simulink model "MBD_W3_Prob3"  (R2020a)
settings: Solver=ode45  StartTime=0.0  StopTime=25  MaxStep=0.01  RelTol=1e-3  AbsTol=1e-6
values from neighbouring files (symbols this model uses):
  g = 9.81    [Prob3.m]
  I = 5    [Prob3.m]
  Kf = 1    [Prob3.m]
  m = 75    [Prob3.m]
  mu = [0 .4 .8 .97 1.0 .98 .96 .94 .92 .9 .88 .855 .83 .81 .79 .77 .75 .73 .72 .71 .7]    [Prob3.m]
  PBmax = 1500    [Prob3.m]
  Rr = 15/12    (= 1.25)    [Prob3.m]
  slip = (0:.05:1.0)    [Prob3.m]
  TB = 0.01    [Prob3.m]
  v0 = 45    [Prob3.m]
settings Model: Creator=Noel Varghese  LastModifiedBy=Noel Varghese

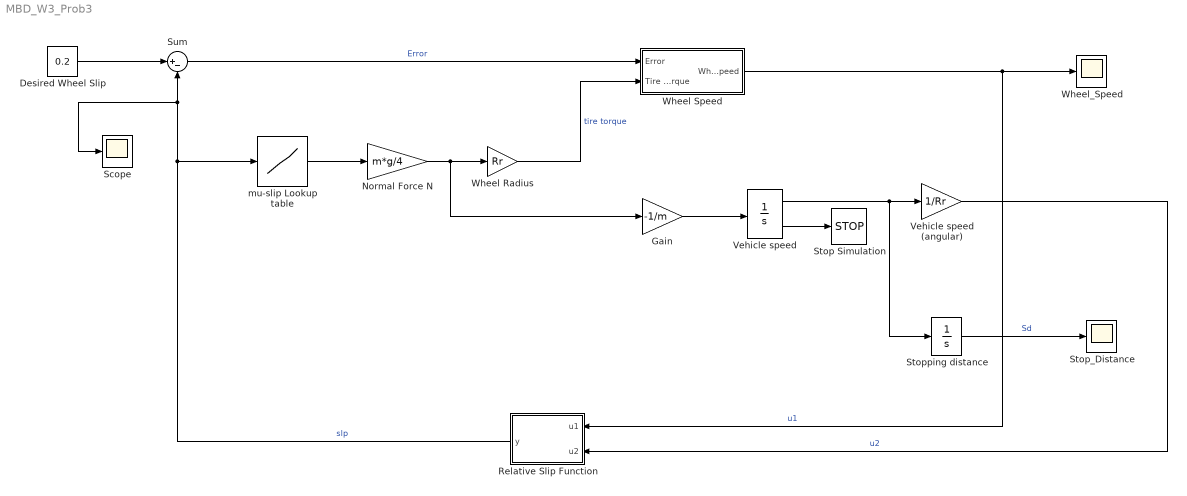
== system MBD_W3_Prob3 ==
  Desired Wheel Slip : Constant  Value=0.2
  Gain : Gain  Gain=-1/m
  Normal Force N : Gain  Gain=m*g/4
  Relative Slip Function : MATLAB Function  TreatAsAtomicUnit=on
  Scope : Scope
  Stop Simulation : Stop
  Stop_Distance : Scope
  Stopping distance : Integrator  UpperSaturationLimit=1000  LowerSaturationLimit=0
  Sum : Sum  Inputs=|+-
  Vehicle speed : Integrator  InitialCondition=v0  LimitOutput=on  UpperSaturationLimit=1000  LowerSaturationLimit=0  ShowSaturationPort=on
  Vehicle speed (angular) : Gain  Gain=1/Rr  SaturateOnIntegerOverflow=on  OutDataTypeStr=Inherit: Same as input  ParamDataTypeStr=Inherit: Same as input
  Wheel Radius : Gain  Gain=Rr
  Wheel Speed : Subsystem
  Wheel_Speed : Scope
  mu-slip Lookup table : Lookup_n-D  NumberOfTableDimensions=1  BreakpointsForDimension1=slip  Table=mu  SaturateOnIntegerOverflow=on  InputSameDT=on
  wires:
  Desired Wheel Slip/1 -> Sum/1
  Sum/1 -> Wheel Speed/1(Error)  "Error"
  mu-slip Lookup table/1 -> Normal Force N/1
  Normal Force N/1 -> Gain/1, Wheel Radius/1
  Wheel Radius/1 -> Wheel Speed/2(Tire Torque)  "tire torque"
  Wheel Speed/1(WheelSpeed) -> Wheel_Speed/1, Relative Slip Function/1(u1)  "u1"
  Gain/1 -> Vehicle speed/1
  Vehicle speed/1 -> Stopping distance/1, Vehicle speed (angular)/1
  Vehicle speed (angular)/1 -> Relative Slip Function/2(u2)  "u2"
  Vehicle speed/2 -> Stop Simulation/1
  Stopping distance/1 -> Stop_Distance/1  "Sd"
  Relative Slip Function/1(y) -> Scope/1, Sum/2, mu-slip Lookup table/1  "slp"

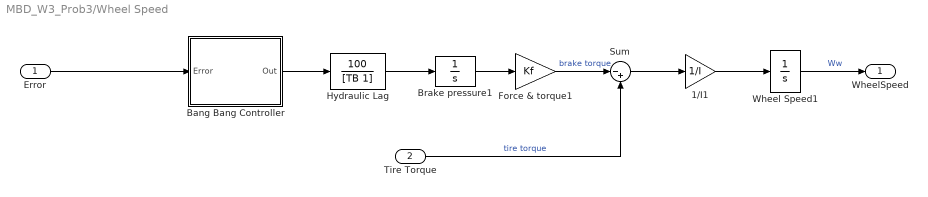
== system MBD_W3_Prob3/Wheel Speed ==
  Error : Inport  SampleTime=0
  Tire Torque : Inport  Port=2
  1/I1 : Gain  Gain=1/I  SaturateOnIntegerOverflow=on  OutDataTypeStr=Inherit: Same as input  ParamDataTypeStr=Inherit: Same as input
  Bang Bang Controller : Subsystem
  Brake pressure1 : Integrator  LimitOutput=on  UpperSaturationLimit=PBmax  LowerSaturationLimit=0
  Force & torque1 : Gain  Gain=Kf  SaturateOnIntegerOverflow=on  OutDataTypeStr=Inherit: Same as input  ParamDataTypeStr=Inherit: Same as input
  "Hydraulic Lag " : TransferFcn  Numerator=[100]  Denominator=[TB 1]
  Sum : Sum  Inputs=|-+  InputSameDT=on  SaturateOnIntegerOverflow=on  OutDataTypeStr=Inherit: Same as first input
  Wheel Speed1 : Integrator  InitialCondition=v0/Rr  LimitOutput=on  UpperSaturationLimit=1000  LowerSaturationLimit=0
  WheelSpeed : Outport  VectorParamsAs1DForOutWhenUnconnected=off
  wires:
  Error/1 -> Bang Bang Controller/1(Error)
  Wheel Speed1/1 -> WheelSpeed/1  "Ww"
  1/I1/1 -> Wheel Speed1/1
  Force & torque1/1 -> Sum/1  "brake torque"
  "Hydraulic Lag "/1 -> Brake pressure1/1
  Brake pressure1/1 -> Force & torque1/1
  Tire Torque/1 -> Sum/2  "tire torque"
  Sum/1 -> 1/I1/1
  Bang Bang Controller/1(Out) -> "Hydraulic Lag "/1

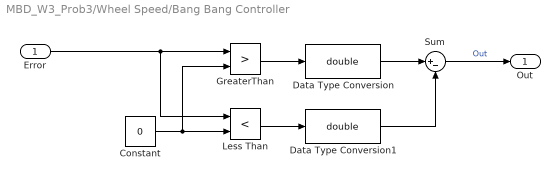
== system MBD_W3_Prob3/Wheel Speed/Bang Bang Controller ==
  Error : Inport  SampleTime=0
  Constant : Constant  Value=0
  Data Type Conversion : DataTypeConversion  OutDataTypeStr=double  RndMeth=Zero
  Data Type Conversion1 : DataTypeConversion  OutDataTypeStr=double  RndMeth=Zero
  GreaterThan : RelationalOperator  Operator=>  OutDataTypeStr=boolean  RndMeth=Simplest
  Less Than : RelationalOperator  Operator=<  OutDataTypeStr=boolean  RndMeth=Simplest
  Sum : Sum  Inputs=|+-
  Out : Outport
  wires:
  GreaterThan/1 -> Data Type Conversion/1
  Error/1 -> Less Than/1, GreaterThan/1
  Data Type Conversion1/1 -> Sum/2
  Constant/1 -> GreaterThan/2, Less Than/2
  Less Than/1 -> Data Type Conversion1/1
  Sum/1 -> Out/1  "Out"
  Data Type Conversion/1 -> Sum/1

== matlab function MBD_W3_Prob3/Relative Slip Function ==
  data: u1 input; y output; u2 input
function y = fcn(u1,u2)
%u1- wheel speed
%u2- angular vehicle speed
y = 1.0-u1/(u2+(u2==0)*eps);
